simulink model "sampleModel1926"  (R2023a)
settings: Solver=VariableStepAuto  StartTime=0.0  StopTime=10.0  RelTol=1e-3
libraries: hdlsllib x2
settings Model: Creator=user1  LastModifiedBy=user1

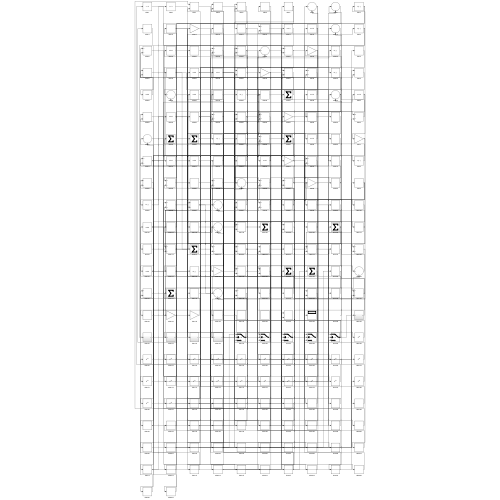
[thumbnail: Simulink's stored preview of the top-level diagram]
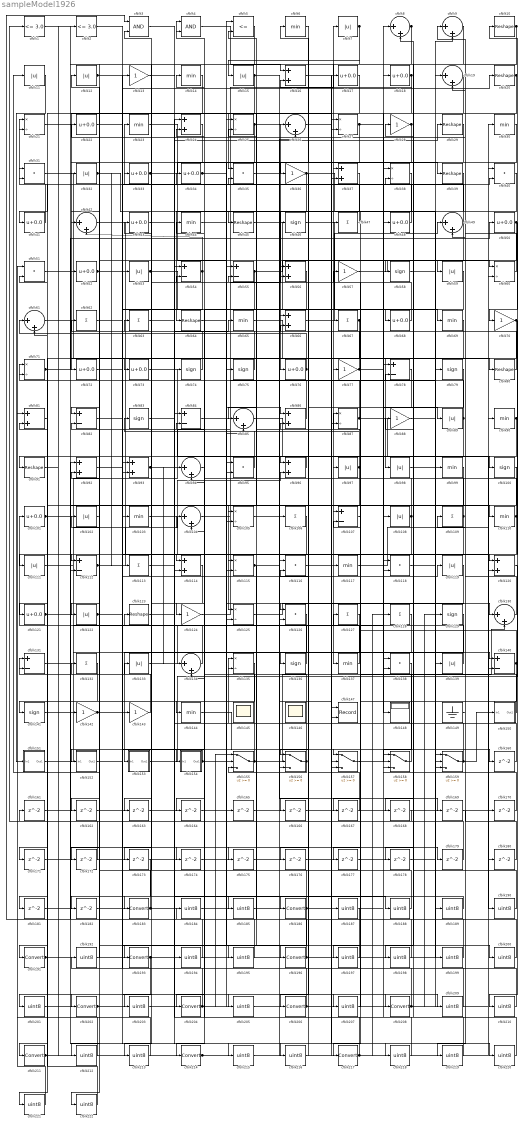
== system sampleModel1926 ==
  cfblk1 : hdlsllib/Logic and Bit Operations/Compare To Constant  relop=<=  const=3.0  OutDataTypeStr=boolean
  cfblk{10,20,29,39,45,64,80,91,123} (9 alike) : Reshape
  cfblk{46,58,74..75,79,83,100,129,136,141} (10 alike) : Signum
  cfblk{17..18,22,33..34,41,43,48,50,52,68,72..73,76,101,121} (16 alike) : Bias  Bias=0.0  SaturateOnIntegerOverflow=off
  cfblk{7,11..12,15,32,53,59,89,97..98,102,108,111,119,122,133,139} (17 alike) : Abs  SaturateOnIntegerOverflow=off
  cfblk{6,14,23,30,44,65,69,90,99,103,110,117,137,144} (14 alike) : MinMax
  cfblk{8..9,19,26,42,49,61,85,94,104,130,134} (12 alike) : Sum  Inputs=|++
  cfblk{21,25,27,38,60,71,87,105,115,125,135} (11 alike) : Product  Inputs=*/  RndMeth=Zero  SaturateOnIntegerOverflow=on
  cfblk{47,62..63,67,106,109,113,127..128,132} (10 alike) : Sum  Inputs=+
  cfblk{54..55,78,82,84,107,112,131,140} (9 alike) : Sum  Inputs=+-
  cfblk{16,24,37,56,66,81,86,92..93,96,114,120} (12 alike) : Sum
  cfblk{31,35,40,51,95,116,118,126,138} (9 alike) : DotProduct  OutDataTypeStr=Inherit: Inherit via internal rule
  cfblk{13,28,36,57,70,77,88,124,142..143} (10 alike) : Gain
  cfblk145 : Scope
      settings: Floating=on
  cfblk146 : Scope
      settings: Floating=on
  cfblk147 : Record  FileSettingsInternal="{\"entries\":[{\"content\":{\"excelSettings\":{\"content\":{},\"type\":\"Streamout.ExcelSettings\"}},\"type\":\"Streamout.FileSettingStorage\",\"uuid\":\"\"}],\"packageUris\":[\"http:\\/\\/schema.mathworks.com\\/mf0\\/streamout_blocks\\/R2020a\"],\"version\":\"1.0\"}"  Layout=[1 1]  SignalsInternal="{\"entries\":[{\"content\":{\"signals\":[{\"content\":{\"blockPath\":[],\"dimensions\":[1],\"domain\":\"\",\"lineColor\":\"#a2142f\",\"plots\":[1],\"port\":1,\"signalID\":5187,\"signalName\":\"XY Graph:1\"},\"type\":\"RecordBlkView.Signal\",\"uuid\":\"\"},{\"content\":{\"blockPath\":[],\"dimensions\":[1],\"domain\":\"\",\"lineColor\":\"#139fff\",\"plots\":[1],\"port\":2,\"signalID\":5190,\"signalName\":\"XY Graph:2\"},\"type\":\"RecordBlkView.Signal\",\"uuid\":\"\"}]},\"type\":\"RecordBlkView.InputSignals\",\"uuid\":\"\"}],\"packageUris\":[\"http:\\/\\/schema.mathworks.com\\/mf0\\/streamout_blocks\\/R2020a\"],\"version\":\"1.0\"}"  VisualizationBindings="{\"xyplotplugin\":{\"info\":[{\"series\":[{\"bindingParametersList\":[{\"parameter\":\"X-Axis\",\"signalID\":5187,\"signalName\":\"XY Graph:1\"},{\"parameter\":\"Y-Axis\",\"signalID\":5190,\"signalName\":\"XY Graph:2\"}],\"seriesID\":22600}],\"subplotID\":1}]}}"  CompatibilityTag=XY  st=-1
  cfblk148 : Display
  cfblk149 : Ground
  cfblk150 : Subsystem
      settings: LibrarySourceBlock=|
      | hdlsllib/Ports &
      | Subsystems/Subsystem
  cfblk151 : Subsystem
      settings: LibrarySourceBlock=|
      | hdlsllib/Ports &
      | Subsystems/Subsystem
  cfblk152 : Subsystem
      settings: LibrarySourceBlock=|
      | hdlsllib/Ports &
      | Subsystems/Subsystem
  cfblk153 : Subsystem
      settings: LibrarySourceBlock=|
      | hdlsllib/Ports &
      | Subsystems/Subsystem
  cfblk154 : Subsystem
      settings: LibrarySourceBlock=|
      | hdlsllib/Ports &
      | Subsystems/Subsystem
  cfblk{155..159} (5 alike) : Switch  SaturateOnIntegerOverflow=off  InputSameDT=off
  cfblk{160..182} (23 alike) : Delay  SampleTime=1
  cfblk{183,186,191,193,196,202,204,206,208,211,214,217} (12 alike) : DataTypeConversion  SaturateOnIntegerOverflow=off  RndMeth=Floor
  cfblk{184..185,187..190,192,194..195,197..201,203,205,207,209..210,212..213,215..216,218..222} (28 alike) : DataTypeConversion  OutDataTypeStr=uint8  SaturateOnIntegerOverflow=off  RndMeth=Floor
  cfblk2 : hdlsllib/Logic and Bit Operations/Compare To Constant  relop=<=  const=3.0  OutDataTypeStr=boolean
  cfblk3 : Logic  AllPortsSameDT=off  OutDataTypeStr=boolean
  cfblk4 : Logic  AllPortsSameDT=off  OutDataTypeStr=boolean
  cfblk5 : RelationalOperator  Operator=<=  OutDataTypeStr=boolean  InputSameDT=off
  wires:
  cfblk42/1 -> cfblk114/1
  cfblk128/1 -> cfblk153/1(In1)
  cfblk15/1 -> cfblk72/1, cfblk147/2
  cfblk47/1 -> cfblk23/1
  cfblk125/1 -> cfblk130/1
  cfblk66/1 -> cfblk49/1
  cfblk91/1 -> cfblk2/1
  cfblk32/1 -> cfblk76/1, cfblk113/1
  cfblk130/1 -> cfblk9/1
  cfblk153/1(Out1) -> cfblk10/1
  cfblk8/1 -> cfblk137/1, cfblk112/2
  cfblk39/1 -> cfblk66/1
  cfblk38/1 -> cfblk64/1
  cfblk48/1 -> cfblk21/1
  cfblk31/1 -> cfblk98/1
  cfblk131/1 -> cfblk136/1
  cfblk55/1 -> cfblk59/1, cfblk154/1(In1)
  cfblk96/1 -> cfblk91/1
  cfblk7/1 -> cfblk15/1, cfblk172/1
  cfblk150/1(Out1) -> cfblk87/1
  cfblk104/1 -> cfblk7/1
  cfblk17/1 -> cfblk35/1
  cfblk80/1 -> cfblk62/1
  cfblk84/1 -> cfblk26/1
  cfblk45/1 -> cfblk77/1
  cfblk56/1 -> cfblk214/1
  cfblk73/1 -> cfblk96/1
  cfblk59/1 -> cfblk144/1
  cfblk109/1 -> cfblk121/1, cfblk6/1, cfblk168/1
  cfblk78/1 -> cfblk217/1
  cfblk12/1 -> cfblk103/1, cfblk69/1
  cfblk63/1 -> cfblk35/2
  cfblk60/1 -> cfblk22/1
  cfblk94/1 -> cfblk124/1
  cfblk53/1 -> cfblk108/1, cfblk179/1
  cfblk99/1 -> cfblk204/1
  cfblk11/1 -> cfblk151/1(In1)
  cfblk9/1 -> cfblk42/1
  cfblk2/1 -> cfblk143/1
  cfblk116/1 -> cfblk208/1
  cfblk138/1 -> cfblk158/2
  cfblk92/1 -> cfblk196/1
  cfblk46/1 -> cfblk68/1
  cfblk25/1 -> cfblk100/1, cfblk213/1
  cfblk74/1 -> cfblk63/1
  cfblk44/1 -> cfblk75/1
  cfblk136/1 -> cfblk84/2
  cfblk3/1 -> cfblk186/1
  cfblk41/1 -> cfblk21/2
  cfblk81/1 -> cfblk211/1
  cfblk29/1 -> cfblk37/1
  cfblk65/1 -> cfblk148/1
  cfblk112/1 -> cfblk96/2, cfblk156/3
  cfblk14/1 -> cfblk32/1
  cfblk33/1 -> cfblk39/1, cfblk29/1
  cfblk133/1 -> cfblk46/1
  cfblk124/1 -> cfblk67/1
  cfblk137/1 -> cfblk101/1
  cfblk134/1 -> cfblk123/1
  cfblk155/1 -> cfblk130/2, cfblk54/2
  cfblk117/1 -> cfblk90/1
  cfblk158/1 -> cfblk57/1
  cfblk82/1 -> cfblk13/1
  cfblk157/1 -> cfblk38/1
  cfblk93/1 -> cfblk9/2, cfblk134/1
  cfblk1/1 -> cfblk27/2
  cfblk143/1 -> cfblk131/1
  cfblk103/1 -> cfblk125/1
  cfblk79/1 -> cfblk126/1
  cfblk151/1(Out1) -> cfblk53/1
  cfblk67/1 -> cfblk111/1, cfblk181/1
  cfblk34/1 -> cfblk47/1, cfblk126/2, cfblk86/1
  cfblk35/1 -> cfblk106/1
  cfblk110/1 -> cfblk28/1, cfblk112/1
  cfblk28/1 -> cfblk105/2, cfblk203/1
  cfblk23/1 -> cfblk125/2
  cfblk57/1 -> cfblk60/1
  cfblk97/1 -> cfblk83/1, cfblk71/2, cfblk171/1
  cfblk77/1 -> cfblk43/1, cfblk89/1
  cfblk68/1 -> cfblk33/1
  cfblk54/1 -> cfblk42/2, cfblk93/2
  cfblk21/1 -> cfblk107/1
  cfblk105/1 -> cfblk157/1
  cfblk121/1 -> cfblk25/1, cfblk175/1
  cfblk76/1 -> cfblk73/1, cfblk61/1
  cfblk37/1 -> cfblk45/1
  cfblk142/1 -> cfblk11/1, cfblk205/1
  cfblk111/1 -> cfblk104/1
  cfblk152/1(Out1) -> cfblk119/1
  cfblk70/1 -> cfblk104/2, cfblk120/1
  cfblk86/1 -> cfblk71/1
  cfblk75/1 -> cfblk4/1
  cfblk10/1 -> cfblk122/1, cfblk178/1
  cfblk126/1 -> cfblk155/2
  cfblk90/1 -> cfblk157/2, cfblk156/1, cfblk162/1
  cfblk135/1 -> cfblk141/1
  cfblk87/1 -> cfblk34/1, cfblk190/1
  cfblk95/1 -> cfblk44/1
  cfblk108/1 -> cfblk14/1, cfblk115/2
  cfblk22/1 -> cfblk110/1
  cfblk20/1 -> cfblk41/1, cfblk85/1
  cfblk154/1(Out1) -> cfblk38/2, cfblk85/2, cfblk152/1(In1)
  cfblk52/1 -> cfblk114/2, cfblk120/2
  cfblk123/1 -> cfblk74/1
  cfblk30/1 -> cfblk202/1
  cfblk141/1 -> cfblk8/1
  cfblk71/1 -> cfblk50/1, cfblk174/1
  cfblk50/1 -> cfblk70/1, cfblk173/1
  cfblk27/1 -> cfblk18/1, cfblk87/2
  cfblk122/1 -> cfblk40/2, cfblk140/1
  cfblk100/1 -> cfblk115/1
  cfblk58/1 -> cfblk79/1
  cfblk89/1 -> cfblk97/1, cfblk61/2
  cfblk115/1 -> cfblk169/1, cfblk185/1
  cfblk36/1 -> cfblk105/1, cfblk139/1, cfblk176/1
  cfblk4/1 -> cfblk16/1
  cfblk62/1 -> cfblk20/1
  cfblk85/1 -> cfblk117/1
  cfblk5/1 -> cfblk183/1
  cfblk24/1 -> cfblk193/1
  cfblk132/1 -> cfblk191/1
  cfblk127/1 -> cfblk206/1
  cfblk139/1 -> cfblk25/2
  cfblk49/1 -> cfblk31/1, cfblk82/1, cfblk58/1
  cfblk102/1 -> cfblk12/1
  cfblk140/1 -> cfblk107/2, cfblk109/1, cfblk177/1
  cfblk159/1 -> cfblk135/1, cfblk94/2, cfblk150/1(In1)
  cfblk101/1 -> cfblk142/1, cfblk65/1
  cfblk18/1 -> cfblk138/2, cfblk16/2
  cfblk149/1 -> cfblk19/2
  cfblk6/1 -> cfblk36/1
  cfblk156/1 -> cfblk155/3, cfblk82/2
  cfblk61/1 -> cfblk80/1
  cfblk98/1 -> cfblk159/1
  cfblk144/1 -> cfblk160/1
  cfblk160/1 -> cfblk84/1
  cfblk161/1 -> cfblk95/1
  cfblk162/1 -> cfblk40/1
  cfblk114/1 -> cfblk163/1
  cfblk163/1 -> cfblk138/1
  cfblk106/1 -> cfblk164/1
  cfblk164/1 -> cfblk55/1
  cfblk165/1 -> cfblk135/2
  cfblk119/1 -> cfblk166/1
  cfblk166/1 -> cfblk60/2
  cfblk107/1 -> cfblk167/1
  cfblk167/1 -> cfblk66/2
  cfblk168/1 -> cfblk1/1
  cfblk170/1 -> cfblk158/1
  cfblk171/1 -> cfblk26/2
  cfblk172/1 -> cfblk31/2
  cfblk175/1 -> cfblk159/2
  cfblk176/1 -> cfblk159/3
  cfblk177/1 -> cfblk158/3
  cfblk178/1 -> cfblk8/2
  cfblk179/1 -> cfblk4/2
  cfblk180/1 -> cfblk49/2
  cfblk181/1 -> cfblk94/1
  cfblk182/1 -> cfblk27/1
  cfblk183/1 -> cfblk102/1, cfblk48/1
  cfblk184/1 -> cfblk5/1
  cfblk185/1 -> cfblk5/2
  cfblk186/1 -> cfblk86/2, cfblk133/1, cfblk222/1
  cfblk16/1 -> cfblk187/1
  cfblk187/1 -> cfblk3/1
  cfblk174/1 -> cfblk188/1
  cfblk188/1 -> cfblk3/2
  cfblk88/1 -> cfblk189/1
  cfblk189/1 -> cfblk182/1
  cfblk190/1 -> cfblk88/1
  cfblk191/1 -> cfblk131/2, cfblk19/1
  cfblk192/1 -> cfblk132/1
  cfblk193/1 -> cfblk165/1, cfblk221/1
  cfblk13/1 -> cfblk194/1
  cfblk194/1 -> cfblk24/1
  cfblk129/1 -> cfblk195/1
  cfblk195/1 -> cfblk24/2
  cfblk196/1 -> cfblk17/1, cfblk55/2
  cfblk40/1 -> cfblk197/1
  cfblk197/1 -> cfblk92/1
  cfblk19/1 -> cfblk198/1
  cfblk198/1 -> cfblk92/2
  cfblk118/1 -> cfblk199/1
  cfblk199/1 -> cfblk161/1
  cfblk64/1 -> cfblk200/1
  cfblk200/1 -> cfblk118/1
  cfblk69/1 -> cfblk201/1
  cfblk201/1 -> cfblk118/2
  cfblk202/1 -> cfblk147/1, cfblk95/2
  cfblk203/1 -> cfblk30/1
  cfblk204/1 -> cfblk192/1, cfblk180/1, cfblk155/1
  cfblk205/1 -> cfblk99/1
  cfblk206/1 -> cfblk140/2, cfblk93/1
  cfblk113/1 -> cfblk207/1
  cfblk207/1 -> cfblk127/1
  cfblk208/1 -> cfblk156/2, cfblk129/1
  cfblk83/1 -> cfblk209/1
  cfblk209/1 -> cfblk116/1
  cfblk120/1 -> cfblk210/1
  cfblk210/1 -> cfblk116/2
  cfblk211/1 -> cfblk37/2, cfblk52/1
  cfblk173/1 -> cfblk212/1
  cfblk212/1 -> cfblk81/1
  cfblk213/1 -> cfblk81/2
  cfblk214/1 -> cfblk170/1, cfblk157/3
  cfblk72/1 -> cfblk215/1
  cfblk215/1 -> cfblk56/1
  cfblk43/1 -> cfblk216/1
  cfblk216/1 -> cfblk56/2
  cfblk217/1 -> cfblk184/1, cfblk134/2, cfblk128/1
  cfblk26/1 -> cfblk218/1
  cfblk218/1 -> cfblk78/1
  cfblk169/1 -> cfblk219/1
  cfblk219/1 -> cfblk78/2
  cfblk51/1 -> cfblk220/1
  cfblk220/1 -> cfblk54/1
  cfblk221/1 -> cfblk51/1
  cfblk222/1 -> cfblk51/2

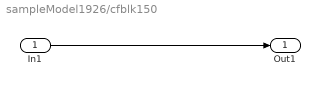
== system sampleModel1926/cfblk150 ==
  In1 : Inport
  Out1 : Outport
  wires:
  In1/1 -> Out1/1

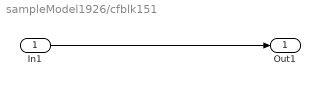
== system sampleModel1926/cfblk151 ==
  In1 : Inport
  Out1 : Outport
  wires:
  In1/1 -> Out1/1

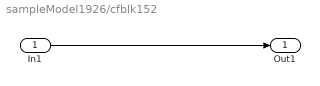
== system sampleModel1926/cfblk152 ==
  In1 : Inport
  Out1 : Outport
  wires:
  In1/1 -> Out1/1

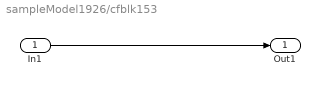
== system sampleModel1926/cfblk153 ==
  In1 : Inport
  Out1 : Outport
  wires:
  In1/1 -> Out1/1

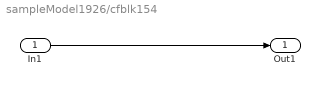
== system sampleModel1926/cfblk154 ==
  In1 : Inport
  Out1 : Outport
  wires:
  In1/1 -> Out1/1
